simulink model "DoorSignal"  (R2022a)
settings: Solver=VariableStepAuto  StartTime=0.0  StopTime=5.1  MinStep=0.001  RelTol=1e-3
values from neighbouring files (symbols this model uses):
  Ddoor = 0.05    [SYDE351Project.m]
  Hdoor = 0.03    [SYDE351Project.m]
  speed = 1    [SYDE351Project.m]
settings Model: Creator=lanam  LastModifiedBy=Bronz

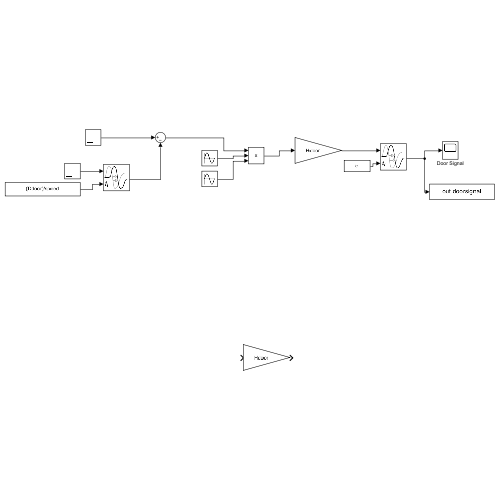
[thumbnail: Simulink's stored preview of the top-level diagram]
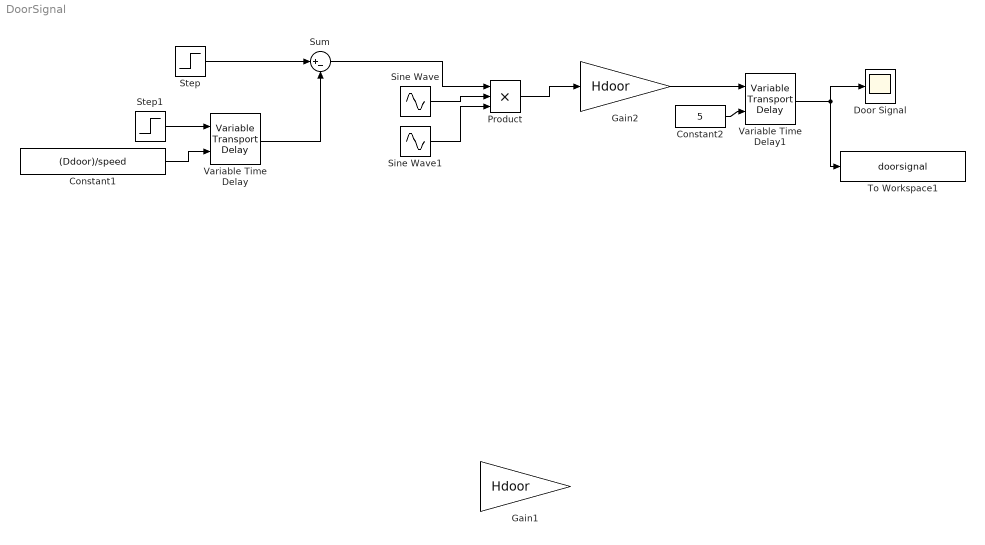
== system DoorSignal ==
  Constant1 : Constant  Value=(Ddoor)/speed
  Constant2 : Constant  Value=5
  Door Signal : Scope
  Gain1 : Gain  Gain=Hdoor
  Gain2 : Gain  Gain=Hdoor
  Product : Product  Inputs=3
  Sine Wave : Sin  Frequency=(pi*speed)/Ddoor  SampleTime=0
  Sine Wave1 : Sin  Frequency=(pi*speed)/Ddoor  SampleTime=0
  Step : Step  Time=0  SampleTime=0
  Step1 : Step  Time=0  SampleTime=0
  Sum : Sum  Inputs=|+-
  To Workspace1 : ToWorkspace  VariableName=doorsignal  SaveFormat=Timeseries  SampleTime=-1
  Variable Time Delay : VariableTransportDelay  VariableDelayType=Variable transport delay  MaximumDelay=100  ZeroDelay=on
  Variable Time Delay1 : VariableTransportDelay  VariableDelayType=Variable transport delay  MaximumDelay=100  ZeroDelay=on
  wires:
  Step1/1 -> Variable Time Delay/1
  Sum/1 -> Product/1
  Variable Time Delay/1 -> Sum/2
  Constant1/1 -> Variable Time Delay/2
  Product/1 -> Gain2/1
  Sine Wave/1 -> Product/2
  Sine Wave1/1 -> Product/3
  Step/1 -> Sum/1
  Gain2/1 -> Variable Time Delay1/1
  Variable Time Delay1/1 -> To Workspace1/1, Door Signal/1
  Constant2/1 -> Variable Time Delay1/2
